simulink model "slexFPGAPredictPreparedExample"  (R2023a)
settings: Solver=FixedStepDiscrete  StartTime=0.0  StopTime=timeVector(end)  FixedStep=stepSize  RelTol=1e-3
values from neighbouring files (symbols this model uses):
  learnerParams = mv(end).Value    [DeployRegressionNeuralNetworkModelToFPGA1.m]
  nnetMdl = fitrnet(trainDataSmall,"Y",LayerSizes=[10,10])    [DeployRegressionNeuralNetworkModelToFPGA1.m]
  X_MAX = minmaxData.X_MAX    [DeployRegressionNeuralNetworkModelToFPGA1.m]    (also in MinMaxVectors.mat = [4.23207255751 5.99961 26.28963])
  X_MIN = minmaxData.X_MIN    [DeployRegressionNeuralNetworkModelToFPGA1.m]    (also in MinMaxVectors.mat = [2.79645479834 -18.0971537397 -10.3047309401])
settings Model: DataTypeOverride=Off  MinMaxOverflowLogging=ForceOff  FPTShortcutValueString='{{},{''BaselineRun'',1,1,1,''BaselineRun'','''',{},''M'','''',''''},{''EmbeddedRun'',1,1,1,''EmbeddedRun'','''',{},''M'','''',''''},{''EmbeddedRun_2'',1,1,1,''EmbeddedRun_2'','''',{},''M'','''',''''},{''EmbeddedRun_3'',1,1,1,''EmbeddedRun_3'','''',{},''M'','''',''''},{''EmbeddedRun_4'',1,1,1,''EmbeddedRun_4'','''',{},''M'','''',''''},{''EmbeddedRun_5'',1,1,1,''EmbeddedRun_5'','''',{},''M'','''',''''},{''EmbeddedRun_6'',1,1,1,''EmbeddedRun_6'','''',{},''M'','''',''''}}'  SimulationMode=accelerator  Creator=The MathWorks, Inc.  LastModifiedBy=The MathWorks, Inc.
settings DataIOCC: SaveTime=off
settings OptimizationCC: BlockReduction=off  ConditionallyExecuteInputs=off  DefaultParameterBehavior=Inlined  InheritOutputTypeSmallerThanSingle=on
settings DebuggingCC: SignalRangeChecking=error  AlgebraicLoopMsg=error  InheritedTsInSrcMsg=none  SingleTaskRateTransMsg=error  IntegerOverflowMsg=none  ParameterDowncastMsg=none  ParameterOverflowMsg=none  ParameterPrecisionLossMsg=none  IntegerSaturationMsg=none
settings HardwareCC: ProdBitPerPointer=32  ProdBitPerSizeT=32  ProdBitPerPtrDiffT=32  ProdLargestAtomicFloat=None  ProdIntDivRoundTo=Undefined  ProdEndianess=Unspecified  ProdWordSize=32  ProdHWDeviceType=ASIC/FPGA->ASIC/FPGA  TargetBitPerLong=64  TargetBitPerPointer=64  TargetBitPerSizeT=64  TargetBitPerPtrDiffT=64  TargetLongLongMode=on  TargetIntDivRoundTo=Zero  TargetEndianess=LittleEndian  TargetWordSize=64  TargetHWDeviceType=Custom Processor->MATLAB Host Computer  ProdEqTarget=off
settings ModelReferenceCC: EnableRefExpFcnMdlSchedulingChecks=on

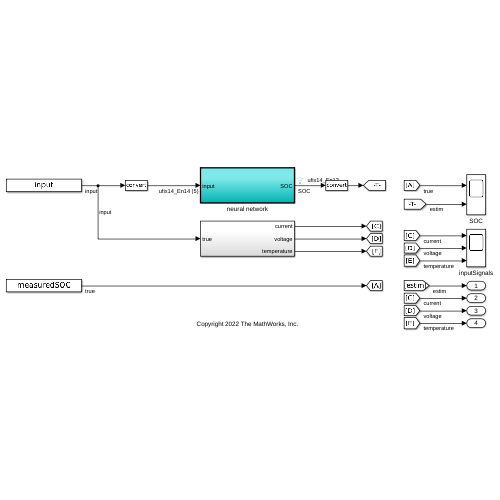
[thumbnail: Simulink's stored preview of the top-level diagram]
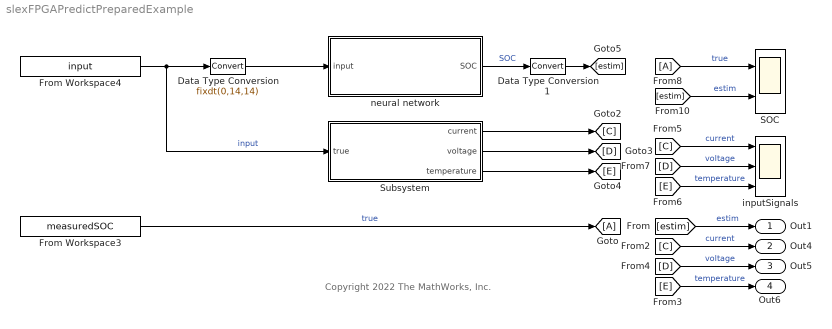
== system slexFPGAPredictPreparedExample ==
  note: Copyright 2022 The MathWorks, Inc.
  Data Type Conversion : DataTypeConversion  OutDataTypeStr=fixdt(0,14,14)  SaturateOnIntegerOverflow=off  RndMeth=Floor
  Data Type Conversion1 : DataTypeConversion  SaturateOnIntegerOverflow=off  RndMeth=Floor
  From Workspace3 : FromWorkspace  VariableName=measuredSOC  SampleTime=-1
  From Workspace4 : FromWorkspace  VariableName=input  SampleTime=-1
  From8 : From
  Goto : Goto
  SOC : Scope  NumInputPorts=2
  Subsystem : Subsystem
  inputSignals : Scope  NumInputPorts=3
  neural network : Subsystem  TreatAsAtomicUnit=on
  Out1 : Outport
  Out4 : Outport  Port=2
  Out5 : Outport  Port=3
  Out6 : Outport  Port=4
  wires:
  Data Type Conversion1/1 -> [estim]
  Data Type Conversion/1 -> neural network/1(input)
  From Workspace4/1 -> Data Type Conversion/1, Subsystem/1(true)  "input"
  [D] -> Out5/1  "voltage"
  [E] -> inputSignals/3  "temperature"
  [estim] -> SOC/2  "estim"
  From8/1 -> SOC/1  "true"
  [C] -> Out4/1  "current"
  [D] -> inputSignals/2  "voltage"
  [C] -> inputSignals/1  "current"
  From Workspace3/1 -> Goto/1  "true"
  neural network/1(SOC) -> Data Type Conversion1/1  "SOC"
  Subsystem/3(temperature) -> [E]
  [estim] -> Out1/1  "estim"
  Subsystem/1(current) -> [C]
  Subsystem/2(voltage) -> [D]
  [E] -> Out6/1  "temperature"

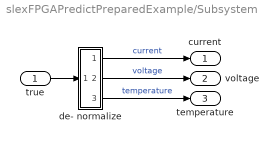
== system slexFPGAPredictPreparedExample/Subsystem ==
  true : Inport
  de- normalize : Subsystem
  current : Outport
  voltage : Outport  Port=2
  temperature : Outport  Port=3
  wires:
  true/1 -> de- normalize/1(u)
  de- normalize/3(T) -> temperature/1  "temperature"
  de- normalize/1(I) -> current/1  "current"
  de- normalize/2(V) -> voltage/1  "voltage"

== system slexFPGAPredictPreparedExample/neural network ==
  input : Inport  OutDataTypeStr=fixdt(0,14,14)  PortDimensions=[5]  SampleTime=10
  RegressionNeuralNetwork Predict : Subsystem  TreatAsAtomicUnit=on  mask(RegressionNeuralNetwork Predict){TrainedLearner=nnetMdl, RndMeth=Floor, SaturateOnIntegerOverflow=off, LockScale=off, OutDataTypeStr=fixdt(0,14,13), OutMin=[], OutMax=[], OutputLayerDataTypeStr=fixdt(1,14,12), OutputLayerOutMin=[], OutputLayerOutMax=[], OutputLayerAdditionDataTypeStr=fixdt(0,14,13), OutputLayerAdditionOutMin=[], OutputLayerAdditionOutMax=[], LayerSelector=Layer 1, Layer1DataTypeStr=fixdt(1,13,10), Layer1OutMin=[], Layer1OutMax=[], Layer1AdditionDataTypeStr=fixdt(1,14,11), Layer1AdditionOutMin=[], Layer1AdditionOutMax=[], Layer2DataTypeStr=fixdt(1,14,11), Layer2OutMin=[], Layer2OutMax=[], Layer2AdditionDataTypeStr=fixdt(1,14,10), Layer2AdditionOutMin=[], Layer2AdditionOutMax=[], Layer3DataTypeStr=Inherit: Inherit via internal rule, Layer3OutMin=[], Layer3OutMax=[], Layer3AdditionDataTypeStr=Inherit: Inherit via internal rule, Layer3AdditionOutMin=[], Layer3AdditionOutMax=[], Layer4DataTypeStr=Inherit: Inherit via internal rule, Layer4OutMin=[], Layer4OutMax=[], Layer4AdditionDataTypeStr=Inherit: Inherit via internal rule, Layer4AdditionOutMin=[], Layer4AdditionOutMax=[], Layer5DataTypeStr=Inherit: Inherit via internal rule, Layer5OutMin=[], Layer5OutMax=[], Layer5AdditionDataTypeStr=Inherit: Inherit via internal rule, Layer5AdditionOutMin=[], Layer5AdditionOutMax=[], Layer6DataTypeStr=Inherit: Inherit via internal rule, Layer6OutMin=[], Layer6OutMax=[], Layer6AdditionDataTypeStr=Inherit: Inherit via internal rule, Layer6AdditionOutMin=[], Layer6AdditionOutMax=[], Layer7DataTypeStr=Inherit: Inherit via internal rule, Layer7OutMin=[], Layer7OutMax=[], Layer7AdditionDataTypeStr=Inherit: Inherit via internal rule, Layer7AdditionOutMin=[], Layer7AdditionOutMax=[], Layer8DataTypeStr=Inherit: Inherit via internal rule, Layer8OutMin=[], Layer8OutMax=[], Layer8AdditionDataTypeStr=Inherit: Inherit via internal rule, Layer8AdditionOutMin=[], Layer8AdditionOutMax=[], Layer9DataTypeStr=Inherit: Inherit via internal rule, Layer9OutMin=[], Layer9OutMax=[], Layer9AdditionDataTypeStr=Inherit: Inherit via internal rule, Layer9AdditionOutMin=[], Layer9AdditionOutMax=[], Layer10DataTypeStr=Inherit: Inherit via internal rule, Layer10OutMin=[], Layer10OutMax=[], Layer10AdditionDataTypeStr=Inherit: Inherit via internal rule, Layer10AdditionOutMin=[], Layer10AdditionOutMax=[], Layer11DataTypeStr=Inherit: Inherit via internal rule, Layer11OutMin=[], Layer11OutMax=[], Layer11AdditionDataTypeStr=Inherit: Inherit via internal rule, Layer11AdditionOutMin=[], Layer11AdditionOutMax=[], StandardizedInputDataTypeStr=fixdt(1,12,8), StandardizedInputOutMin=[], StandardizedInputOutMax=[], NumHiddenLayers=1}
      mask prompts: TrainedLearner "Select trained machine learning model"; RndMeth "Integer rounding mode"; SaturateOnIntegerOverflow "Simulink:blkprm_prompts:AllBlksSaturate"; LockScale "Simulink:blkprm_prompts:LockScale"; OutDataTypeStr "Output data type"; OutputLayerDataTypeStr "Output layer data type"; OutputLayerAdditionDataTypeStr "Output layer addition data type"; LayerSelector "Select a layer"; Layer1DataTypeStr "Layer 1 data type"; Layer1AdditionDataTypeStr "Layer 1 addition data type"; Layer2DataTypeStr "Layer 2 data type"; Layer2AdditionDataTypeStr "Layer 2 addition data type"; Layer3DataTypeStr "Layer 3 data type"; Layer3AdditionDataTypeStr "Layer 3 addition data type"; Layer4DataTypeStr "Layer 4 data type"; Layer4AdditionDataTypeStr "Layer 4 addition data type"; Layer5DataTypeStr "Layer 5 data type"; Layer5AdditionDataTypeStr "Layer 5 addition data type"; Layer6DataTypeStr "Layer 6 data type"; Layer6AdditionDataTypeStr "Layer 6 addition data type"; Layer7DataTypeStr "Layer 7 data type"; Layer7AdditionDataTypeStr "Layer 7 addition data type"; Layer8DataTypeStr "Layer 8 data type"; Layer8AdditionDataTypeStr "Layer 8 addition data type"; Layer9DataTypeStr "Layer 9 data type"; Layer9AdditionDataTypeStr "Layer 9 addition data type"; Layer10DataTypeStr "Layer 10 data type"; Layer10AdditionDataTypeStr "Layer 10 addition data type"; Layer11DataTypeStr "Additional layer(s) data type"; Layer11AdditionDataTypeStr "Additional layer(s) addition data type"; StandardizedInputDataTypeStr "Standardized input data type"; NumHiddenLayers "Number of hidden layers"
      mask help: Predict responses using neural networks
      mask init:
      | dlgParamsIn.ModelName = TrainedLearner;
      | dlgParamsIn.NumHiddenLayers = NumHiddenLayers;
      | 
      | [learnerParams,dlgParamsOut] = classregblks.nnet.maskInitialization(gcbh,dlgParamsIn,'regr');
      | NumHiddenLayers = dlgParamsOut.NumHiddenLayers;
      | 
      | % Avoid storing the dlg variables twice in the MaskWSVariables 
      | clear dlgParamsIn dlgParamsOut;
      settings: LibrarySourceBlock=statsLibrary/Regression/RegressionNeuralNetwork Predict
      mask Help: helpview(fullfile(docroot,'stats','stats.map'),'RegressionNeuralNetworkPredict')
      mask TypeOptions RndMeth: getScore/hiddenLayers/hiddenLayer1/RndMeth | getScore/outputLayer/Add/RndMeth | getScore/outputLayer/Data Type Conversion/RndMeth | getScore/outputLayer/Product/RndMeth | standardize/standardize/Add/RndMeth | standardize/standardize/Divide/RndMeth
      mask TypeOptions SaturateOnIntegerOverflow: getScore/hiddenLayers/hiddenLayer1/SaturateOnIntegerOverflow | getScore/outputLayer/Add/SaturateOnIntegerOverflow | getScore/outputLayer/Data Type Conversion/SaturateOnIntegerOverflow | getScore/outputLayer/Product/SaturateOnIntegerOverflow | standardize/standardize/Add/SaturateOnIntegerOverflow | standardize/standardize/Divide/SaturateOnIntegerOverflow
      mask TypeOptions LockScale: x/LockScale | getScore/X/LockScale | getScore/hiddenLayers/X/LockScale | getScore/hiddenLayers/hiddenLayer1/LockScale | getScore/hiddenLayers/L/LockScale | getScore/outputLayer/X/LockScale | getScore/outputLayer/Add/LockScale | getScore/outputLayer/Data Type Conversion/LockScale | getScore/outputLayer/Product/LockScale | getScore/outputLayer/bias/LockScale | getScore/outputLayer/weights/LockScale | getScore/outputLayer/L/LockScale | getScore/yfit/LockScale | standardize/X/LockScale | standardize/passthrough/X/LockScale | standardize/passthrough/Xnorm/LockScale | standardize/standardize/X/LockScale | standardize/standardize/Add/LockScale | standardize/standardize/Divide/LockScale | standardize/standardize/Mu/LockScale | standardize/standardize/Sigma/LockScale | standardize/standardize/Xnorm/LockScale | standardize/Xnorm/LockScale | yfit/LockScale
      mask TypeOptions LayerSelector: Layer 1 | Layer 2 | All layers
      mask Callback LayerSelector: classregblks.nnet.callbackLayerVisibility(gcbh)
      mask DialogControl DescTrainedModel Prompt: Trained Machine Learning Model
      mask DialogControl ButtonInfoRefresh Prompt: Refresh
      mask DialogControl ButtonInfoRefresh Callback: classregblks.callbacks.refreshLearnerInfo(gcbh,'nnet','regr')
      mask DialogControl DescLayerSizes Prompt: Layer sizes: [10,10]
      mask DialogControl DescActivations Prompt: Activations: relu
      mask DialogControl DescStandardize Prompt: Standardized: false
      mask DialogControl tabMain Prompt: Main
      mask DialogControl tabDataTypes Prompt: Data Types
      mask DialogControl tabFixedPointOpParams Prompt: Fixed-Point Operational Parameters
      mask DialogControl SaturateOnIntegerOverflow Prompt: Saturate on integer overflow
      mask DialogControl LockScale Prompt: Lock output data type setting against changes by the fixed-point tools
      mask DialogControl txtDataType Prompt: Simulink:dialog:DataTypeColumnLabel
      mask DialogControl txtMinimum Prompt: Simulink:dialog:MinimumColumnLabel
      mask DialogControl txtMaximum Prompt: Simulink:dialog:MaximumColumnLabel
      mask DialogControl grpExtraDataTypes Prompt: Additional data types
  Transpose : Math  Operator=transpose  OutDataTypeStr=double
  SOC : Outport  OutDataTypeStr=fixdt(0,14,13)  SampleTime=10
  wires:
  input/1 -> Transpose/1
  RegressionNeuralNetwork Predict/1(yfit) -> SOC/1
  Transpose/1 -> RegressionNeuralNetwork Predict/1(x)

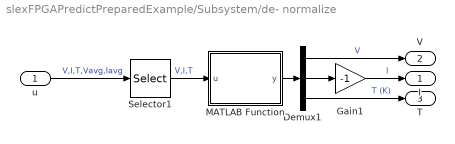
== system slexFPGAPredictPreparedExample/Subsystem/de- normalize ==
  u : Inport
  Demux1 : Demux  Outputs=3
  Gain1 : Gain  Gain=-1
  MATLAB Function : MATLAB Function  TreatAsAtomicUnit=on
  Selector1 : Selector  InputPortWidth=5  IndexOptions=Index vector (dialog)  Indices=[1 2 3]  OutputSizes=1
  I : Outport
  V : Outport  Port=2
  T : Outport  Port=3
  wires:
  Gain1/1 -> I/1  "I"
  Selector1/1 -> MATLAB Function/1(u)  "V,I,T"
  Demux1/2 -> Gain1/1
  Demux1/1 -> V/1  "V"
  Demux1/3 -> T/1  "T (K)"
  MATLAB Function/1(y) -> Demux1/1
  u/1 -> Selector1/1  "V,I,T,Vavg,Iavg"

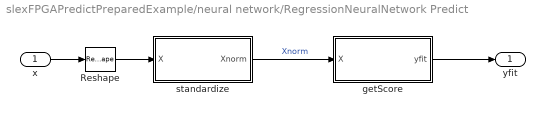
== system slexFPGAPredictPreparedExample/neural network/RegressionNeuralNetwork Predict ==
  x : Inport
  Reshape : Reshape  OutputDimensionality=Row vector (2-D)
  getScore : Subsystem
  standardize : Subsystem  Variant=on
  yfit : Outport  OutMin=OutMin  OutMax=OutMax  OutDataTypeStr=OutDataTypeStr  VectorParamsAs1DForOutWhenUnconnected=off
  wires:
  getScore/1(yfit) -> yfit/1
  standardize/1(Xnorm) -> getScore/1(X)  "Xnorm"
  x/1 -> Reshape/1
  Reshape/1 -> standardize/1(X)

== system slexFPGAPredictPreparedExample/neural network/RegressionNeuralNetwork Predict/getScore ==
  X : Inport
  hiddenLayers : Subsystem
  outputLayer : Subsystem
  yfit : Outport
  wires:
  outputLayer/1(L) -> yfit/1
  hiddenLayers/1(L) -> outputLayer/1(X)
  X/1 -> hiddenLayers/1(X)

== system slexFPGAPredictPreparedExample/neural network/RegressionNeuralNetwork Predict/standardize ==
  X : Inport  PortDimensions=[1,learnerParams.NumPredictors]
  passthrough : Subsystem  VariantControl=~learnerParams.doNormalize
  standardize : Subsystem  VariantControl=learnerParams.doNormalize
  Xnorm : Outport

== system slexFPGAPredictPreparedExample/neural network/RegressionNeuralNetwork Predict/getScore/hiddenLayers ==
  X : Inport
  hiddenLayer1 : Subsystem  VariantControl=Relu  mask(Neural Network Layer){LearnerParams=learnerParams, LayerWeights=learnerParams.PredictWeights{1}, LayerBias=learnerParams.Bias{1}, LayerActivation=relu, RndMeth=Floor, SaturateOnIntegerOverflow=off, LockScale=off, LayerProductDataTypeStr=Layer1DataTypeStr, LayerProductOutMin=Layer1OutMin, LayerProductOutMax=Layer1OutMax, LayerAdditionDataTypeStr=Layer1AdditionDataTypeStr, AdditionOutMin=Layer1AdditionOutMin, AdditionOutMax=Layer1AdditionOutMax, LayerActivationDataTypeStr=Inherit: auto, ActivationOutMin=[], ActivationOutMax=[]}
      mask prompts: LearnerParams "Learner Parameters"; LayerWeights "Weights"; LayerBias "Bias"; LayerActivation "Activation"; RndMeth "Integer rounding mode"; SaturateOnIntegerOverflow "Simulink:blkprm_prompts:AllBlksSaturate"; LockScale "Simulink:blkprm_prompts:LockScale"; LayerProductDataTypeStr "Multiplier data type"; LayerAdditionDataTypeStr "Addition data type"; LayerActivationDataTypeStr "Activation data type"
      mask help: This block implements a fully-connected layer for a neural network
      settings: LibrarySourceBlock=sharedstatsblks/hiddenLayer
      mask TypeOptions LayerWeights: weights/Value
      mask TypeOptions LayerBias: bias/Value
      mask TypeOptions LayerActivation: Activation/LabelModeActiveChoice
      mask TypeOptions RndMeth: Activation/relu/MinMax/RndMeth | Activation/sigmoid/Data Type Conversion/RndMeth | Activation/sigmoid/Tanh Variant/Approximate/Source/Data Type Conversion/RndMeth | Activation/sigmoid/Tanh Variant/Approximate/Source/LUT/RndMeth | Activation/sigmoid/Tanh Variant/Original/DTCIn_1/RndMeth | Activation/sigmoid/Tanh Variant/Original/Data Type Conversion1/RndMeth | Activation/tanh/Tanh Variant/Approximate/Source/Data Type Conversion/RndMeth | Activation/tanh/Tanh Variant/Approximate/Source/LUT/RndMeth | Activation/tanh/Tanh Variant/Original/DTCIn_1/RndMeth | Activation/tanh/Tanh Variant/Original/Data Type Conversion1/RndMeth | Add/RndMeth | Product/RndMeth
      mask TypeOptions SaturateOnIntegerOverflow: Activation/relu/MinMax/SaturateOnIntegerOverflow | Activation/sigmoid/Bias/SaturateOnIntegerOverflow | Activation/sigmoid/Data Type Conversion/SaturateOnIntegerOverflow | Activation/sigmoid/Tanh Variant/Approximate/Source/Data Type Conversion/SaturateOnIntegerOverflow | Activation/sigmoid/Tanh Variant/Approximate/Source/LUT/SaturateOnIntegerOverflow | Activation/sigmoid/Tanh Variant/Original/DTCIn_1/SaturateOnIntegerOverflow | Activation/sigmoid/Tanh Variant/Original/Data Type Conversion1/SaturateOnIntegerOverflow | Activation/tanh/Tanh Variant/Approximate/Source/Data Type Conversion/SaturateOnIntegerOverflow | Activation/tanh/Tanh Variant/Approximate/Source/LUT/SaturateOnIntegerOverflow | Activation/tanh/Tanh Variant/Original/DTCIn_1/SaturateOnIntegerOverflow | Activation/tanh/Tanh Variant/Original/Data Type Conversion1/SaturateOnIntegerOverflow | Add/SaturateOnIntegerOverflow | Product/SaturateOnIntegerOverflow
      mask TypeOptions LockScale: Lin/LockScale | Activation/In1/LockScale | Activation/none/In1/LockScale | Activation/none/L/LockScale | Activation/relu/In1/LockScale | Activation/relu/Constant/LockScale | Activation/relu/MinMax/LockScale | Activation/relu/L/LockScale | Activation/sigmoid/In1/LockScale | Activation/sigmoid/Data Type Conversion/LockScale | Activation/sigmoid/Tanh Variant/In1/LockScale | Activation/sigmoid/Tanh Variant/Approximate/In1/LockScale | Activation/sigmoid/Tanh Variant/Approximate/Source/In1/LockScale | Activation/sigmoid/Tanh Variant/Approximate/Source/Data Type Conversion/LockScale | Activation/sigmoid/Tanh Variant/Approximate/Source/LUT/LockScale | Activation/sigmoid/Tanh Variant/Approximate/Source/Out1/LockScale | Activation/sigmoid/Tanh Variant/Approximate/Out1/LockScale | Activation/sigmoid/Tanh Variant/Original/In1/LockScale | Activation/sigmoid/Tanh Variant/Original/DTCIn_1/LockScale | Activation/sigmoid/Tanh Variant/Original/Data Type Conversion1/LockScale | Activation/sigmoid/Tanh Variant/Original/Out1/LockScale | Activation/sigmoid/Tanh Variant/Out1/LockScale | Activation/sigmoid/L/LockScale | Activation/tanh/In1/LockScale | Activation/tanh/Tanh Variant/In1/LockScale | Activation/tanh/Tanh Variant/Approximate/In1/LockScale | Activation/tanh/Tanh Variant/Approximate/Source/In1/LockScale | Activation/tanh/Tanh Variant/Approximate/Source/Data Type Conversion/LockScale | Activation/tanh/Tanh Variant/Approximate/Source/LUT/LockScale | Activation/tanh/Tanh Variant/Approximate/Source/Out1/LockScale | Activation/tanh/Tanh Variant/Approximate/L/LockScale | Activation/tanh/Tanh Variant/Original/In1/LockScale | Activation/tanh/Tanh Variant/Original/DTCIn_1/LockScale | Activation/tanh/Tanh Variant/Original/Data Type Conversion1/LockScale | Activation/tanh/Tanh Variant/Original/L/LockScale | Activation/tanh/Tanh Variant/L/LockScale | Activation/tanh/L/LockScale | Activation/L/LockScale | Add/LockScale | Product/LockScale | bias/LockScale | weights/LockScale | Lout/LockScale
      mask TypeOptions LayerProductDataTypeStr: Product/OutDataTypeStr
      mask TypeOptions LayerProductOutMin: Product/OutMin
      mask TypeOptions LayerProductOutMax: Product/OutMax
      mask TypeOptions LayerAdditionDataTypeStr: Add/OutDataTypeStr
      mask TypeOptions AdditionOutMin: Add/OutMin
      mask TypeOptions AdditionOutMax: Add/OutMax
      mask TypeOptions LayerActivationDataTypeStr: Lout/OutDataTypeStr
      mask TypeOptions ActivationOutMin: Lout/OutMin
      mask TypeOptions ActivationOutMax: Lout/OutMax
      mask DialogControl tabFixedPointOpParams Prompt: Fixed-Point Operational Parameters
      mask DialogControl SaturateOnIntegerOverflow Prompt: Saturate on integer overflow
      mask DialogControl LockScale Prompt: Lock output data type setting against changes by the fixed-point tools
      mask DialogControl txtDataType Prompt: Simulink:dialog:DataTypeColumnLabel
      mask DialogControl txtMinimum Prompt: Simulink:dialog:MinimumColumnLabel
      mask DialogControl txtMaximum Prompt: Simulink:dialog:MaximumColumnLabel
  hiddenLayer2 : Subsystem  VariantControl=Relu  mask(Neural Network Layer){LearnerParams=learnerParams, LayerWeights=learnerParams.PredictWeights{2}, LayerBias=learnerParams.Bias{2}, LayerActivation=relu, RndMeth=Floor, SaturateOnIntegerOverflow=off, LockScale=off, LayerProductDataTypeStr=Layer2DataTypeStr, LayerProductOutMin=Layer2OutMin, LayerProductOutMax=Layer2OutMax, LayerAdditionDataTypeStr=Layer2AdditionDataTypeStr, AdditionOutMin=Layer2AdditionOutMin, AdditionOutMax=Layer2AdditionOutMax, LayerActivationDataTypeStr=Inherit: auto, ActivationOutMin=[], ActivationOutMax=[]}
      mask prompts: LearnerParams "Learner Parameters"; LayerWeights "Weights"; LayerBias "Bias"; LayerActivation "Activation"; RndMeth "Integer rounding mode"; SaturateOnIntegerOverflow "Simulink:blkprm_prompts:AllBlksSaturate"; LockScale "Simulink:blkprm_prompts:LockScale"; LayerProductDataTypeStr "Multiplier data type"; LayerAdditionDataTypeStr "Addition data type"; LayerActivationDataTypeStr "Activation data type"
      mask help: This block implements a fully-connected layer for a neural network
      settings: LibrarySourceBlock=sharedstatsblks/hiddenLayer
      mask TypeOptions LayerWeights: weights/Value
      mask TypeOptions LayerBias: bias/Value
      mask TypeOptions LayerActivation: Activation/LabelModeActiveChoice
      mask TypeOptions RndMeth: Activation/relu/MinMax/RndMeth | Activation/sigmoid/Data Type Conversion/RndMeth | Activation/sigmoid/Tanh Variant/Approximate/Source/Data Type Conversion/RndMeth | Activation/sigmoid/Tanh Variant/Approximate/Source/LUT/RndMeth | Activation/sigmoid/Tanh Variant/Original/DTCIn_1/RndMeth | Activation/sigmoid/Tanh Variant/Original/Data Type Conversion1/RndMeth | Activation/tanh/Tanh Variant/Approximate/Source/Data Type Conversion/RndMeth | Activation/tanh/Tanh Variant/Approximate/Source/LUT/RndMeth | Activation/tanh/Tanh Variant/Original/DTCIn_1/RndMeth | Activation/tanh/Tanh Variant/Original/Data Type Conversion1/RndMeth | Add/RndMeth | Product/RndMeth
      mask TypeOptions SaturateOnIntegerOverflow: Activation/relu/MinMax/SaturateOnIntegerOverflow | Activation/sigmoid/Bias/SaturateOnIntegerOverflow | Activation/sigmoid/Data Type Conversion/SaturateOnIntegerOverflow | Activation/sigmoid/Tanh Variant/Approximate/Source/Data Type Conversion/SaturateOnIntegerOverflow | Activation/sigmoid/Tanh Variant/Approximate/Source/LUT/SaturateOnIntegerOverflow | Activation/sigmoid/Tanh Variant/Original/DTCIn_1/SaturateOnIntegerOverflow | Activation/sigmoid/Tanh Variant/Original/Data Type Conversion1/SaturateOnIntegerOverflow | Activation/tanh/Tanh Variant/Approximate/Source/Data Type Conversion/SaturateOnIntegerOverflow | Activation/tanh/Tanh Variant/Approximate/Source/LUT/SaturateOnIntegerOverflow | Activation/tanh/Tanh Variant/Original/DTCIn_1/SaturateOnIntegerOverflow | Activation/tanh/Tanh Variant/Original/Data Type Conversion1/SaturateOnIntegerOverflow | Add/SaturateOnIntegerOverflow | Product/SaturateOnIntegerOverflow
      mask TypeOptions LockScale: Lin/LockScale | Activation/In1/LockScale | Activation/none/In1/LockScale | Activation/none/L/LockScale | Activation/relu/In1/LockScale | Activation/relu/Constant/LockScale | Activation/relu/MinMax/LockScale | Activation/relu/L/LockScale | Activation/sigmoid/In1/LockScale | Activation/sigmoid/Data Type Conversion/LockScale | Activation/sigmoid/Tanh Variant/In1/LockScale | Activation/sigmoid/Tanh Variant/Approximate/In1/LockScale | Activation/sigmoid/Tanh Variant/Approximate/Source/In1/LockScale | Activation/sigmoid/Tanh Variant/Approximate/Source/Data Type Conversion/LockScale | Activation/sigmoid/Tanh Variant/Approximate/Source/LUT/LockScale | Activation/sigmoid/Tanh Variant/Approximate/Source/Out1/LockScale | Activation/sigmoid/Tanh Variant/Approximate/Out1/LockScale | Activation/sigmoid/Tanh Variant/Original/In1/LockScale | Activation/sigmoid/Tanh Variant/Original/DTCIn_1/LockScale | Activation/sigmoid/Tanh Variant/Original/Data Type Conversion1/LockScale | Activation/sigmoid/Tanh Variant/Original/Out1/LockScale | Activation/sigmoid/Tanh Variant/Out1/LockScale | Activation/sigmoid/L/LockScale | Activation/tanh/In1/LockScale | Activation/tanh/Tanh Variant/In1/LockScale | Activation/tanh/Tanh Variant/Approximate/In1/LockScale | Activation/tanh/Tanh Variant/Approximate/Source/In1/LockScale | Activation/tanh/Tanh Variant/Approximate/Source/Data Type Conversion/LockScale | Activation/tanh/Tanh Variant/Approximate/Source/LUT/LockScale | Activation/tanh/Tanh Variant/Approximate/Source/Out1/LockScale | Activation/tanh/Tanh Variant/Approximate/L/LockScale | Activation/tanh/Tanh Variant/Original/In1/LockScale | Activation/tanh/Tanh Variant/Original/DTCIn_1/LockScale | Activation/tanh/Tanh Variant/Original/Data Type Conversion1/LockScale | Activation/tanh/Tanh Variant/Original/L/LockScale | Activation/tanh/Tanh Variant/L/LockScale | Activation/tanh/L/LockScale | Activation/L/LockScale | Add/LockScale | Product/LockScale | bias/LockScale | weights/LockScale | Lout/LockScale
      mask TypeOptions LayerProductDataTypeStr: Product/OutDataTypeStr
      mask TypeOptions LayerProductOutMin: Product/OutMin
      mask TypeOptions LayerProductOutMax: Product/OutMax
      mask TypeOptions LayerAdditionDataTypeStr: Add/OutDataTypeStr
      mask TypeOptions AdditionOutMin: Add/OutMin
      mask TypeOptions AdditionOutMax: Add/OutMax
      mask TypeOptions LayerActivationDataTypeStr: Lout/OutDataTypeStr
      mask TypeOptions ActivationOutMin: Lout/OutMin
      mask TypeOptions ActivationOutMax: Lout/OutMax
      mask DialogControl tabFixedPointOpParams Prompt: Fixed-Point Operational Parameters
      mask DialogControl SaturateOnIntegerOverflow Prompt: Saturate on integer overflow
      mask DialogControl LockScale Prompt: Lock output data type setting against changes by the fixed-point tools
      mask DialogControl txtDataType Prompt: Simulink:dialog:DataTypeColumnLabel
      mask DialogControl txtMinimum Prompt: Simulink:dialog:MinimumColumnLabel
      mask DialogControl txtMaximum Prompt: Simulink:dialog:MaximumColumnLabel
  L : Outport
  wires:
  hiddenLayer2/1(Lout) -> L/1
  hiddenLayer1/1(Lout) -> hiddenLayer2/1(Lin)
  X/1 -> hiddenLayer1/1(Lin)

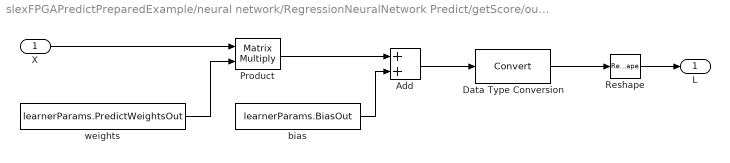
== system slexFPGAPredictPreparedExample/neural network/RegressionNeuralNetwork Predict/getScore/outputLayer ==
  X : Inport
  Add : Sum  OutMin=OutputLayerAdditionOutMin  OutMax=OutputLayerAdditionOutMax  OutDataTypeStr=OutputLayerAdditionDataTypeStr
  Data Type Conversion : DataTypeConversion  SaturateOnIntegerOverflow=off  RndMeth=Floor
  Product : Product  Multiplication=Matrix(*)  OutMin=OutputLayerOutMin  OutMax=OutputLayerOutMax  OutDataTypeStr=OutputLayerDataTypeStr
  Reshape : Reshape
  bias : Constant  Value=learnerParams.BiasOut
  weights : Constant  Value=learnerParams.PredictWeightsOut
  L : Outport
  wires:
  Data Type Conversion/1 -> Reshape/1
  Reshape/1 -> L/1
  Add/1 -> Data Type Conversion/1
  bias/1 -> Add/2
  X/1 -> Product/1
  Product/1 -> Add/1
  weights/1 -> Product/2

== system slexFPGAPredictPreparedExample/neural network/RegressionNeuralNetwork Predict/standardize/passthrough ==
  X : Inport
  Xnorm : Outport
  wires:
  X/1 -> Xnorm/1

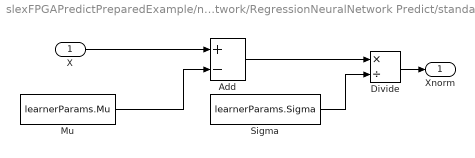
== system slexFPGAPredictPreparedExample/neural network/RegressionNeuralNetwork Predict/standardize/standardize ==
  X : Inport
  Add : Sum  Inputs=+-
  Divide : Product  Inputs=*/  OutMin=StandardizedInputOutMin  OutMax=StandardizedInputOutMax  OutDataTypeStr=StandardizedInputDataTypeStr
  Mu : Constant  Value=learnerParams.Mu  VectorParams1D=off
  Sigma : Constant  Value=learnerParams.Sigma
  Xnorm : Outport  VectorParamsAs1DForOutWhenUnconnected=off
  wires:
  X/1 -> Add/1
  Divide/1 -> Xnorm/1
  Add/1 -> Divide/1
  Sigma/1 -> Divide/2
  Mu/1 -> Add/2

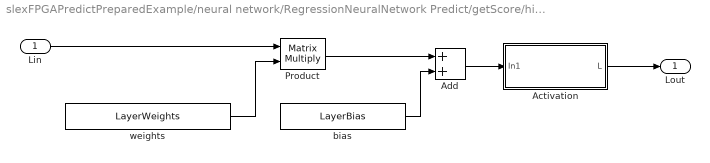
== system slexFPGAPredictPreparedExample/neural network/RegressionNeuralNetwork Predict/getScore/hiddenLayers/hiddenLayer1 ==
  Lin : Inport
  Activation : Subsystem  Variant=on  VariantControlMode=label  LabelModeActiveChoice=relu
  Add : Sum  OutMin=AdditionOutMin  OutMax=AdditionOutMax  OutDataTypeStr=Layer1AdditionDataTypeStr
  Product : Product  Multiplication=Matrix(*)  OutMin=LayerProductOutMin  OutMax=LayerProductOutMax  OutDataTypeStr=Layer1DataTypeStr
  bias : Constant  Value=LayerBias
  weights : Constant  Value=LayerWeights  VectorParams1D=off
  Lout : Outport  OutMin=ActivationOutMin  OutMax=ActivationOutMax
  wires:
  weights/1 -> Product/2
  Add/1 -> Activation/1(In1)
  Product/1 -> Add/1
  Activation/1(L) -> Lout/1
  Lin/1 -> Product/1
  bias/1 -> Add/2

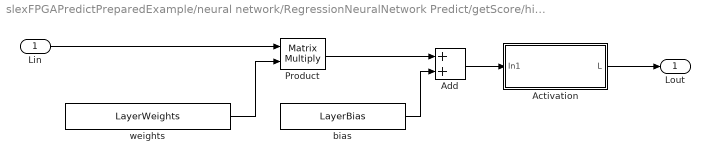
== system slexFPGAPredictPreparedExample/neural network/RegressionNeuralNetwork Predict/getScore/hiddenLayers/hiddenLayer2 ==
  Lin : Inport
  Activation : Subsystem  Variant=on  VariantControlMode=label  LabelModeActiveChoice=relu
  Add : Sum  OutMin=AdditionOutMin  OutMax=AdditionOutMax  OutDataTypeStr=Layer2AdditionDataTypeStr
  Product : Product  Multiplication=Matrix(*)  OutMin=LayerProductOutMin  OutMax=LayerProductOutMax  OutDataTypeStr=Layer2DataTypeStr
  bias : Constant  Value=LayerBias
  weights : Constant  Value=LayerWeights  VectorParams1D=off
  Lout : Outport  OutMin=ActivationOutMin  OutMax=ActivationOutMax
  wires:
  weights/1 -> Product/2
  Add/1 -> Activation/1(In1)
  Product/1 -> Add/1
  Activation/1(L) -> Lout/1
  Lin/1 -> Product/1
  bias/1 -> Add/2

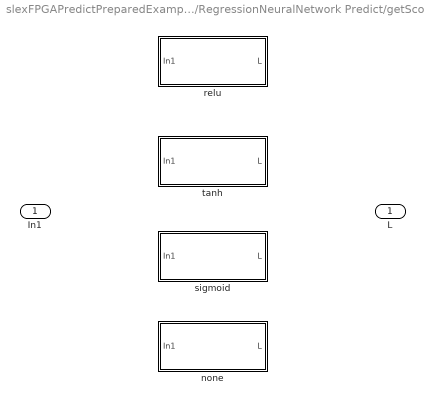
== system slexFPGAPredictPreparedExample/neural network/RegressionNeuralNetwork Predict/getScore/hiddenLayers/hiddenLayer1/Activation ==
  In1 : Inport
  none : Subsystem  VariantControl=none
  relu : Subsystem  VariantControl=relu
  sigmoid : Subsystem  VariantControl=sigmoid
  tanh : Subsystem  VariantControl=tanh
  L : Outport

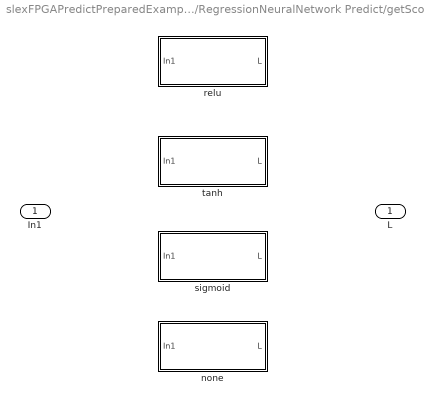
== system slexFPGAPredictPreparedExample/neural network/RegressionNeuralNetwork Predict/getScore/hiddenLayers/hiddenLayer2/Activation ==
  In1 : Inport
  none : Subsystem  VariantControl=none
  relu : Subsystem  VariantControl=relu
  sigmoid : Subsystem  VariantControl=sigmoid
  tanh : Subsystem  VariantControl=tanh
  L : Outport

== system slexFPGAPredictPreparedExample/neural network/RegressionNeuralNetwork Predict/getScore/hiddenLayers/hiddenLayer1/Activation/none ==
  In1 : Inport
  L : Outport
  wires:
  In1/1 -> L/1

== system slexFPGAPredictPreparedExample/neural network/RegressionNeuralNetwork Predict/getScore/hiddenLayers/hiddenLayer1/Activation/relu ==
  In1 : Inport
  Constant : Constant  Value=0  OutDataTypeStr=Inherit: Inherit via back propagation
  MinMax : MinMax  Function=max  Inputs=2  OutDataTypeStr=Inherit: Inherit via back propagation
  L : Outport
  wires:
  In1/1 -> MinMax/1
  MinMax/1 -> L/1
  Constant/1 -> MinMax/2

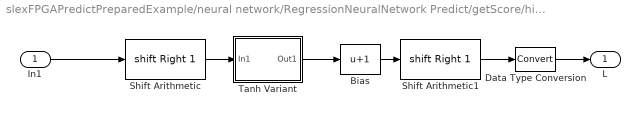
== system slexFPGAPredictPreparedExample/neural network/RegressionNeuralNetwork Predict/getScore/hiddenLayers/hiddenLayer1/Activation/sigmoid ==
  In1 : Inport
  Bias : Bias  Bias=1  SaturateOnIntegerOverflow=off
  Data Type Conversion : DataTypeConversion  SaturateOnIntegerOverflow=off  RndMeth=Floor
  Shift Arithmetic : ArithShift  BitShiftNumber=1  BitShiftDirection=Right
  Shift Arithmetic1 : ArithShift  BitShiftNumber=1  BitShiftDirection=Right
  Tanh Variant : Subsystem  Variant=on
  L : Outport
  wires:
  Data Type Conversion/1 -> L/1
  In1/1 -> Shift Arithmetic/1
  Shift Arithmetic1/1 -> Data Type Conversion/1
  Tanh Variant/1(Out1) -> Bias/1
  Shift Arithmetic/1 -> Tanh Variant/1(In1)
  Bias/1 -> Shift Arithmetic1/1

== system slexFPGAPredictPreparedExample/neural network/RegressionNeuralNetwork Predict/getScore/hiddenLayers/hiddenLayer1/Activation/tanh ==
  In1 : Inport
  Tanh Variant : Subsystem  Variant=on
  L : Outport
  wires:
  Tanh Variant/1(L) -> L/1
  In1/1 -> Tanh Variant/1(In1)

== system slexFPGAPredictPreparedExample/neural network/RegressionNeuralNetwork Predict/getScore/hiddenLayers/hiddenLayer2/Activation/none ==
  In1 : Inport
  L : Outport
  wires:
  In1/1 -> L/1

== system slexFPGAPredictPreparedExample/neural network/RegressionNeuralNetwork Predict/getScore/hiddenLayers/hiddenLayer2/Activation/relu ==
  In1 : Inport
  Constant : Constant  Value=0  OutDataTypeStr=Inherit: Inherit via back propagation
  MinMax : MinMax  Function=max  Inputs=2  OutDataTypeStr=Inherit: Inherit via back propagation
  L : Outport
  wires:
  In1/1 -> MinMax/1
  MinMax/1 -> L/1
  Constant/1 -> MinMax/2

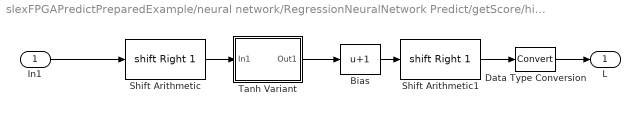
== system slexFPGAPredictPreparedExample/neural network/RegressionNeuralNetwork Predict/getScore/hiddenLayers/hiddenLayer2/Activation/sigmoid ==
  In1 : Inport
  Bias : Bias  Bias=1  SaturateOnIntegerOverflow=off
  Data Type Conversion : DataTypeConversion  SaturateOnIntegerOverflow=off  RndMeth=Floor
  Shift Arithmetic : ArithShift  BitShiftNumber=1  BitShiftDirection=Right
  Shift Arithmetic1 : ArithShift  BitShiftNumber=1  BitShiftDirection=Right
  Tanh Variant : Subsystem  Variant=on
  L : Outport
  wires:
  Data Type Conversion/1 -> L/1
  In1/1 -> Shift Arithmetic/1
  Shift Arithmetic1/1 -> Data Type Conversion/1
  Tanh Variant/1(Out1) -> Bias/1
  Shift Arithmetic/1 -> Tanh Variant/1(In1)
  Bias/1 -> Shift Arithmetic1/1

== system slexFPGAPredictPreparedExample/neural network/RegressionNeuralNetwork Predict/getScore/hiddenLayers/hiddenLayer2/Activation/tanh ==
  In1 : Inport
  Tanh Variant : Subsystem  Variant=on
  L : Outport
  wires:
  Tanh Variant/1(L) -> L/1
  In1/1 -> Tanh Variant/1(In1)

== system slexFPGAPredictPreparedExample/neural network/RegressionNeuralNetwork Predict/getScore/hiddenLayers/hiddenLayer1/Activation/sigmoid/Tanh Variant ==
  In1 : Inport
  Approximate : Subsystem  Tag=Approximate  VariantControl=LearnerParams.IsFxpt
  Original : Subsystem  Tag=Original  VariantControl=~LearnerParams.IsFxpt
  Out1 : Outport

== system slexFPGAPredictPreparedExample/neural network/RegressionNeuralNetwork Predict/getScore/hiddenLayers/hiddenLayer1/Activation/tanh/Tanh Variant ==
  In1 : Inport
  Approximate : Subsystem  Tag=Approximate  VariantControl=LearnerParams.IsFxpt
  Original : Subsystem  Tag=Original  VariantControl=~LearnerParams.IsFxpt
  L : Outport

== system slexFPGAPredictPreparedExample/neural network/RegressionNeuralNetwork Predict/getScore/hiddenLayers/hiddenLayer2/Activation/sigmoid/Tanh Variant ==
  In1 : Inport
  Approximate : Subsystem  Tag=Approximate  VariantControl=LearnerParams.IsFxpt
  Original : Subsystem  Tag=Original  VariantControl=~LearnerParams.IsFxpt
  Out1 : Outport

== system slexFPGAPredictPreparedExample/neural network/RegressionNeuralNetwork Predict/getScore/hiddenLayers/hiddenLayer2/Activation/tanh/Tanh Variant ==
  In1 : Inport
  Approximate : Subsystem  Tag=Approximate  VariantControl=LearnerParams.IsFxpt
  Original : Subsystem  Tag=Original  VariantControl=~LearnerParams.IsFxpt
  L : Outport

== system slexFPGAPredictPreparedExample/neural network/RegressionNeuralNetwork Predict/getScore/hiddenLayers/hiddenLayer1/Activation/sigmoid/Tanh Variant/Approximate ==
  In1 : Inport
  Source : Subsystem  Description=This block was created using function approximation.
  Out1 : Outport
  wires:
  Source/1(Out1) -> Out1/1
  In1/1 -> Source/1(In1)

== system slexFPGAPredictPreparedExample/neural network/RegressionNeuralNetwork Predict/getScore/hiddenLayers/hiddenLayer1/Activation/sigmoid/Tanh Variant/Original ==
  In1 : Inport
  DTCIn_1 : DataTypeConversion  OutDataTypeStr=double  SaturateOnIntegerOverflow=off  RndMeth=Floor
  Data Type Conversion1 : DataTypeConversion  SaturateOnIntegerOverflow=off  RndMeth=Floor
  Source : Trigonometry  Operator=tanh
  Out1 : Outport
  wires:
  Source/1 -> Data Type Conversion1/1
  In1/1 -> DTCIn_1/1
  DTCIn_1/1 -> Source/1
  Data Type Conversion1/1 -> Out1/1

== system slexFPGAPredictPreparedExample/neural network/RegressionNeuralNetwork Predict/getScore/hiddenLayers/hiddenLayer1/Activation/tanh/Tanh Variant/Approximate ==
  In1 : Inport
  Source : Subsystem  Description=This block was created using function approximation.
  L : Outport
  wires:
  In1/1 -> Source/1(In1)
  Source/1(Out1) -> L/1

== system slexFPGAPredictPreparedExample/neural network/RegressionNeuralNetwork Predict/getScore/hiddenLayers/hiddenLayer1/Activation/tanh/Tanh Variant/Original ==
  In1 : Inport
  DTCIn_1 : DataTypeConversion  OutDataTypeStr=double  SaturateOnIntegerOverflow=off  RndMeth=Floor
  Data Type Conversion1 : DataTypeConversion  SaturateOnIntegerOverflow=off  RndMeth=Floor
  Source : Trigonometry  Operator=tanh
  L : Outport
  wires:
  Data Type Conversion1/1 -> L/1
  DTCIn_1/1 -> Source/1
  In1/1 -> DTCIn_1/1
  Source/1 -> Data Type Conversion1/1

== system slexFPGAPredictPreparedExample/neural network/RegressionNeuralNetwork Predict/getScore/hiddenLayers/hiddenLayer2/Activation/sigmoid/Tanh Variant/Approximate ==
  In1 : Inport
  Source : Subsystem  Description=This block was created using function approximation.
  Out1 : Outport
  wires:
  Source/1(Out1) -> Out1/1
  In1/1 -> Source/1(In1)

== system slexFPGAPredictPreparedExample/neural network/RegressionNeuralNetwork Predict/getScore/hiddenLayers/hiddenLayer2/Activation/sigmoid/Tanh Variant/Original ==
  In1 : Inport
  DTCIn_1 : DataTypeConversion  OutDataTypeStr=double  SaturateOnIntegerOverflow=off  RndMeth=Floor
  Data Type Conversion1 : DataTypeConversion  SaturateOnIntegerOverflow=off  RndMeth=Floor
  Source : Trigonometry  Operator=tanh
  Out1 : Outport
  wires:
  Source/1 -> Data Type Conversion1/1
  In1/1 -> DTCIn_1/1
  DTCIn_1/1 -> Source/1
  Data Type Conversion1/1 -> Out1/1

== system slexFPGAPredictPreparedExample/neural network/RegressionNeuralNetwork Predict/getScore/hiddenLayers/hiddenLayer2/Activation/tanh/Tanh Variant/Approximate ==
  In1 : Inport
  Source : Subsystem  Description=This block was created using function approximation.
  L : Outport
  wires:
  In1/1 -> Source/1(In1)
  Source/1(Out1) -> L/1

== system slexFPGAPredictPreparedExample/neural network/RegressionNeuralNetwork Predict/getScore/hiddenLayers/hiddenLayer2/Activation/tanh/Tanh Variant/Original ==
  In1 : Inport
  DTCIn_1 : DataTypeConversion  OutDataTypeStr=double  SaturateOnIntegerOverflow=off  RndMeth=Floor
  Data Type Conversion1 : DataTypeConversion  SaturateOnIntegerOverflow=off  RndMeth=Floor
  Source : Trigonometry  Operator=tanh
  L : Outport
  wires:
  Data Type Conversion1/1 -> L/1
  DTCIn_1/1 -> Source/1
  In1/1 -> DTCIn_1/1
  Source/1 -> Data Type Conversion1/1

== system slexFPGAPredictPreparedExample/neural network/RegressionNeuralNetwork Predict/getScore/hiddenLayers/hiddenLayer1/Activation/sigmoid/Tanh Variant/Approximate/Source ==
  In1 : Inport
  Data Type Conversion : DataTypeConversion  SaturateOnIntegerOverflow=off  RndMeth=Floor
  LUT : Lookup_n-D  NumberOfTableDimensions=1  LookupTableObject=FunctionApproximation_LUTObject_20210329T002800015  BreakpointsForDimension1=LearnerParams.TanhLUT.BreakPoints  BreakpointsForDimension3=[5, 7]  BreakpointsForDimension1DataTypeStr=numerictype(1,8,5)  Table=LearnerParams.TanhLUT.TableData  TableDataTypeStr=numerictype(1,16,15)  ExtrapMethod=Clip  UseLastTableValue=on  InternalRulePriority=Speed  OutDataTypeStr=numerictype(1,16,14)  InputSameDT=off
  Out1 : Outport
  wires:
  Data Type Conversion/1 -> Out1/1
  In1/1 -> LUT/1
  LUT/1 -> Data Type Conversion/1

== system slexFPGAPredictPreparedExample/neural network/RegressionNeuralNetwork Predict/getScore/hiddenLayers/hiddenLayer1/Activation/tanh/Tanh Variant/Approximate/Source ==
  In1 : Inport
  Data Type Conversion : DataTypeConversion  SaturateOnIntegerOverflow=off  RndMeth=Floor
  LUT : Lookup_n-D  NumberOfTableDimensions=1  LookupTableObject=FunctionApproximation_LUTObject_20210329T002800015  BreakpointsForDimension1=LearnerParams.TanhLUT.BreakPoints  BreakpointsForDimension3=[5, 7]  BreakpointsForDimension1DataTypeStr=numerictype(1,8,5)  Table=LearnerParams.TanhLUT.TableData  TableDataTypeStr=numerictype(1,16,15)  ExtrapMethod=Clip  UseLastTableValue=on  InternalRulePriority=Speed  OutDataTypeStr=numerictype(1,16,15)  InputSameDT=off
  Out1 : Outport
  wires:
  Data Type Conversion/1 -> Out1/1
  LUT/1 -> Data Type Conversion/1
  In1/1 -> LUT/1

== system slexFPGAPredictPreparedExample/neural network/RegressionNeuralNetwork Predict/getScore/hiddenLayers/hiddenLayer2/Activation/sigmoid/Tanh Variant/Approximate/Source ==
  In1 : Inport
  Data Type Conversion : DataTypeConversion  SaturateOnIntegerOverflow=off  RndMeth=Floor
  LUT : Lookup_n-D  NumberOfTableDimensions=1  LookupTableObject=FunctionApproximation_LUTObject_20210329T002800015  BreakpointsForDimension1=LearnerParams.TanhLUT.BreakPoints  BreakpointsForDimension3=[5, 7]  BreakpointsForDimension1DataTypeStr=numerictype(1,8,5)  Table=LearnerParams.TanhLUT.TableData  TableDataTypeStr=numerictype(1,16,15)  ExtrapMethod=Clip  UseLastTableValue=on  InternalRulePriority=Speed  OutDataTypeStr=numerictype(1,16,14)  InputSameDT=off
  Out1 : Outport
  wires:
  Data Type Conversion/1 -> Out1/1
  In1/1 -> LUT/1
  LUT/1 -> Data Type Conversion/1

== system slexFPGAPredictPreparedExample/neural network/RegressionNeuralNetwork Predict/getScore/hiddenLayers/hiddenLayer2/Activation/tanh/Tanh Variant/Approximate/Source ==
  In1 : Inport
  Data Type Conversion : DataTypeConversion  SaturateOnIntegerOverflow=off  RndMeth=Floor
  LUT : Lookup_n-D  NumberOfTableDimensions=1  LookupTableObject=FunctionApproximation_LUTObject_20210329T002800015  BreakpointsForDimension1=LearnerParams.TanhLUT.BreakPoints  BreakpointsForDimension3=[5, 7]  BreakpointsForDimension1DataTypeStr=numerictype(1,8,5)  Table=LearnerParams.TanhLUT.TableData  TableDataTypeStr=numerictype(1,16,15)  ExtrapMethod=Clip  UseLastTableValue=on  InternalRulePriority=Speed  OutDataTypeStr=numerictype(1,16,15)  InputSameDT=off
  Out1 : Outport
  wires:
  Data Type Conversion/1 -> Out1/1
  LUT/1 -> Data Type Conversion/1
  In1/1 -> LUT/1

== matlab function slexFPGAPredictPreparedExample/Subsystem/de- normalize/MATLAB Function ==
  data: u input; y output; X_MAX parameter; X_MIN parameter
function y = fcn(u, X_MAX, X_MIN)
y = (X_MAX-X_MIN).*u+X_MIN;
y(3) = y(3) + 273.15; % convert to K
